simulink model "kers_discharge_22_6_update_2019a"  (R2019b)
settings: Solver=ode4  StartTime=0.0  StopTime=50  FixedStep=0.01  RelTol=1e-3
values from neighbouring files (symbols this model uses):
  d = 0.5*rho*Cx*Sf    (= 0.81)    [Data.m]
  Jeq_v = M*Rw^2    (= 83.853)    [Data.m]
  Jf = 1/2*(Rf^2*Mf)    (= 0.025)    [Data.m]
  k = 4/3*mi_d*R_clutch    (= 0.096)    [Data.m]
  Rw = 0.33    [Data.m]
  tau1 = 1/3.08    (= 0.324675324675)    [Data.m]
  tau2 = 1/2.18    (= 0.45871559633)    [Data.m]
  tau3 = 1/1.63    (= 0.613496932515)    [Data.m]
  tau4 = 1/1.29    (= 0.77519379845)    [Data.m]
  tau5 = 1/1.03    (= 0.970873786408)    [Data.m]
  tau6 = 1/0.84    (= 1.19047619048)    [Data.m]
  tau7 = 1/0.69    (= 1.44927536232)    [Data.m]
  tau_max = 2.5    [Data.m]
  tau_min = 0.4    [Data.m]
  tau_trasm_discharge = 1/(tauk_discharge*tauf)    (= 4.77818181818)    [Data.m]
  tauf = 1/4.38    (= 0.228310502283)    [Data.m]
  tauk_discharge = 11*tauk_charge    (= 0.916666666667)    [Data.m]
  Tmax = 240    [Data.m]
  V1max = tauf*tau1*Rw*Wmax    (= 23.0528375734)    [Data.m]
  V2max = tauf*tau2*Rw*Wmax    (= 32.5700640945)    [Data.m]
  V3max = tauf*tau3*Rw*Wmax    (= 43.5599630221)    [Data.m]
  V4max = tauf*tau4*Rw*Wmax    (= 55.0408835085)    [Data.m]
  V5max = tauf*tau5*Rw*Wmax    (= 68.9346987631)    [Data.m]
  V6max = tauf*tau6*Rw*Wmax    (= 84.5270711024)    [Data.m]
  wf_max = 64500/9.55    (= 6753.92670157)    [Data.m]
libraries: simulink x3
settings Model: Creator=andre  LastModifiedBy=andre
settings SolverCC: ZeroCrossControl=DisableAll
settings SFSimCC: CustomCodeUndefinedFunction=UseInterfaceOnly

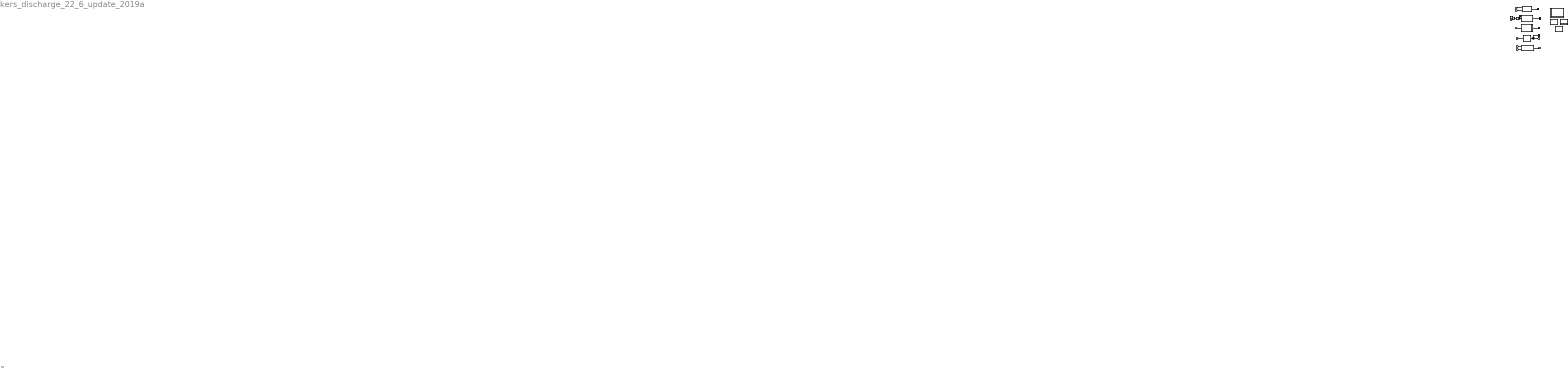
== system kers_discharge_22_6_update_2019a ==
  note: KERS DISCHARGE
  note: v [km/h]
  note: w_f [rpm]
  note: v [km/h]
  note: tau
  Compute Force control for clutch engagement : Subsystem
  Compute Paero : Subsystem
  Compute Pclutch : Subsystem
  Compute Torque to the wheels : Subsystem
  Constant : Constant  Value=Tmax  SampleTime=-1
  From6 : From  Commented=on  GotoTag=Teq  TagVisibility=global
  GearBox : Subsystem
      mask Display: image("GearBox.jpg")
  KERS : Subsystem
      mask Display: image('KERS.jpg'); % Use "Edit Image" on toolstrip to change.
  Product : Product
  Scope{,1..4} (5 alike) : Scope
  Torotrak : Subsystem
      mask Display: image('Torotrak.jpg'); % Use "Edit Image" on toolstrip to change.
  Torque ICE : Subsystem
      mask Display: image("ICE.jpg")
  Vehicle Dynamics : Subsystem
      mask Display: image('Ferrari.jpg'); % Use "Edit Image" on toolstrip to change.
  tag scope: Te=global, taugb=global
  wires:
  [wr] -> Torotrak/1(In1)
  [wf] -> Torotrak/2(In2)
  Torotrak/1(Out1) -> Scope3/1
  [Teq] -> Vehicle Dynamics/1(In1)
  Vehicle Dynamics/1(Out1) -> Scope/1
  KERS/1(Out1) -> Scope1/1
  [v] -> GearBox/1(In1)
  GearBox/1(Out1) -> [taugb], Scope2/1
  [v] -> Torque ICE/1(In1)
  [taugb] -> Torque ICE/2(In2)
  Torque ICE/1(Out1) -> [Te]
  Product/1 -> Scope4/1, KERS/1(In1)
  Constant/1 -> Product/1
  [logic] -> Product/2

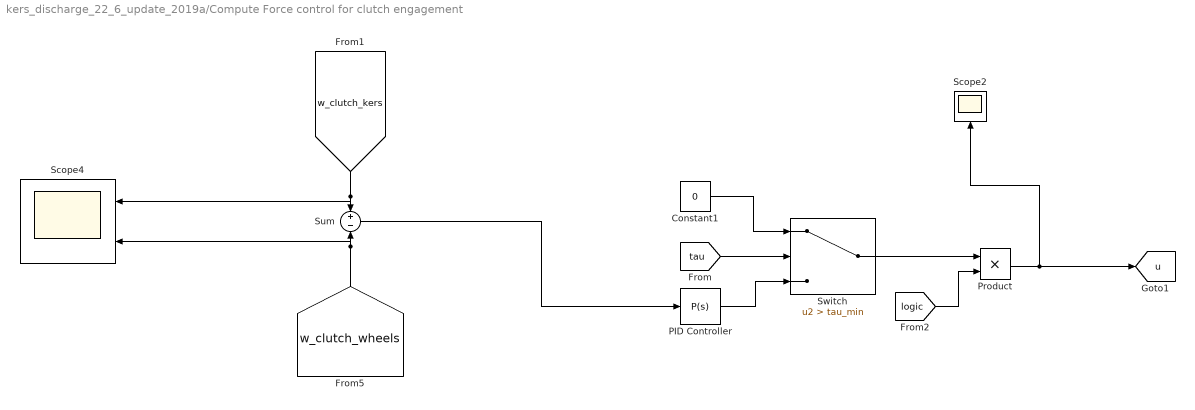
== system kers_discharge_22_6_update_2019a/Compute Force control for clutch engagement ==
  Constant1 : Constant  Value=0  SampleTime=-1
  PID Controller : simulink/Continuous/PID Controller  Controller=P  Form=Parallel  TimeDomain=Continuous-time  SampleTime=-1  IntegratorMethod=Forward Euler  FilterMethod=Forward Euler  ControllerParametersSource=internal  P=0.5  I=1  D=4  UseFilter=on  N=100  TunerSelectOption=Transfer Function Based (PID Tuner App)  InitialConditionSource=internal  InitialConditionForIntegrator=0  InitialConditionForFilter=0  DifferentiatorICPrevScaledInput=0  ExternalReset=none  TrackingMode=off  Kt=1  LimitOutput=off  UpperSaturationLimit=inf  LowerSaturationLimit=-inf  LinearizeAsGain=on  AntiWindupMode=none  Kb=1  POutMin=[]  POutMax=[]  IOutMin=[]  IOutMax=[]  DOutMin=[]  DOutMax=[]  NOutMin=[]  NOutMax=[]  SumOutMin=[]  SumOutMax=[]  SaturationOutMin=[]  SaturationOutMax=[]  PParamMin=[]  PParamMax=[]  IParamMin=[]  IParamMax=[]  DParamMin=[]  DParamMax=[]  NParamMin=[]  NParamMax=[]  KbParamMin=[]  KbParamMax=[]  KtParamMin=[]  KtParamMax=[]  KbOutMin=[]  KbOutMax=[]  KtOutMin=[]  KtOutMax=[]  IntegratorOutMin=[]  IntegratorOutMax=[]  FilterOutMin=[]  FilterOutMax=[]  SumI1OutMin=[]  SumI1OutMax=[]  SumI2OutMin=[]  SumI2OutMax=[]  SumI3OutMin=[]  SumI3OutMax=[]  SumI4OutMin=[]  SumI4OutMax=[]  SumDOutMin=[]  SumDOutMax=[]  DifferentiatorOutMin=[]  DifferentiatorOutMax=[]  FilterDiffOutCoefMin=[]  FilterDiffOutCoefMax=[]  ReciprocalOutMin=[]  ReciprocalOutMax=[]  SumDenOutMin=[]  SumDenOutMax=[]  SumNumOutMin=[]  SumNumOutMax=[]  DivideOutMin=[]  DivideOutMax=[]  IntegratorContinuousStateAttributes=''  IntegratorStateMustResolveToSignalObject=off  IntegratorRTWStateStorageClass=Auto  FilterContinuousStateAttributes=''  FilterStateMustResolveToSignalObject=off  FilterRTWStateStorageClass=Auto  ParallelPVariant=InternalParameters  IdealPVariant=Disabled  IVariant=Disabled  DVariant=Disabled  IntegratorVariant=Disabled  SatVariant=Disabled  AWVariant=Disabled  PCopyVariant=Disabled  TRVariant=Disabled  FdbkBlocksVariant=Forward  IdealPFdbkVariant=Disabled  SatFdbkVariant=Disabled  DerivativeFilterVariant=Disabled  NVariant=Disabled  NCopyVariant=Disabled_SignalSpec  FilterICVariant=Disabled  IntegratorICVariant=Disabled  ExternalResetVariant=Disabled  TRSumVariant=Passthrough  SumFdbkVariant=Disabled  SumVariant=Passthrough_P
  Product : Product
  Scope2 : Scope
  Scope4 : Scope  NumInputPorts=2
  Sum : Sum  Inputs=+-
  Switch : Switch  Criteria=u2 > Threshold  Threshold=tau_min
  tag scope: u=global
  wires:
  [tau] -> Switch/2
  [w_clutch_kers] -> Scope4/1, Sum/1
  [w_clutch_wheels] -> Scope4/2, Sum/2
  Constant1/1 -> Switch/1
  PID Controller/1 -> Switch/3
  Switch/1 -> Product/1
  [logic] -> Product/2
  Product/1 -> Scope2/1, [u]
  Sum/1 -> PID Controller/1

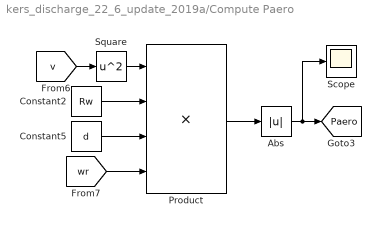
== system kers_discharge_22_6_update_2019a/Compute Paero ==
  Abs : Abs  ZeroCross=off
  Constant2 : Constant  Value=Rw
  Constant5 : Constant  Value=d
  Product : Product  Inputs=4
  Scope : Scope
  Square : Math  Operator=square  SignedPower=on  SaturateOnIntegerOverflow=on
  tag scope: Paero=global
  wires:
  Square/1 -> Product/1
  Constant5/1 -> Product/3
  [wr] -> Product/4
  [v] -> Square/1
  Constant2/1 -> Product/2
  Product/1 -> Abs/1
  Abs/1 -> Scope/1, [Paero]

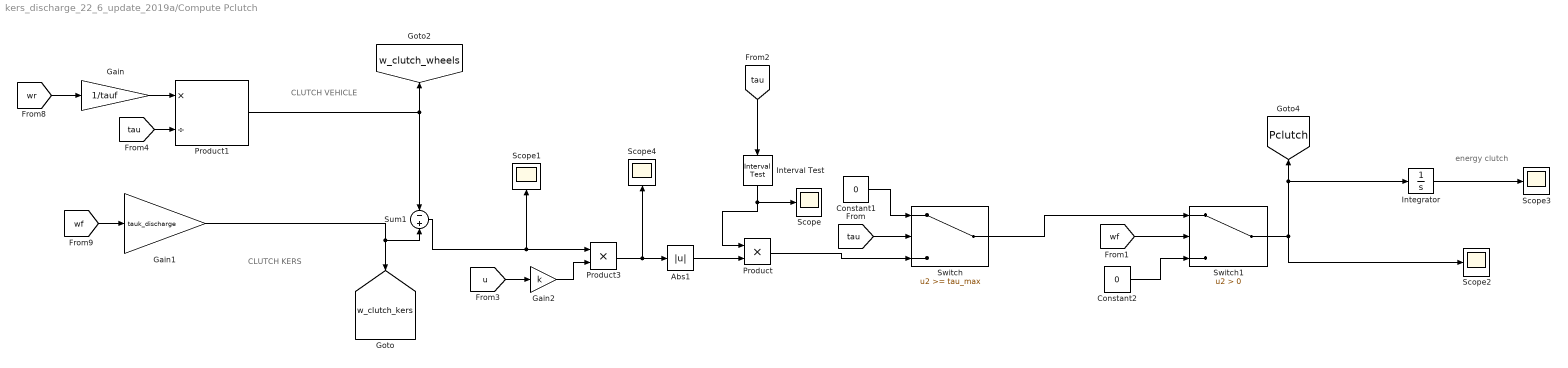
== system kers_discharge_22_6_update_2019a/Compute Pclutch ==
  note: energy clutch
  note: CLUTCH VEHICLE
  note: CLUTCH KERS
  Abs1 : Abs  ZeroCross=off
  Constant1 : Constant  Value=0
  Constant2 : Constant  Value=0
  Gain : Gain  Gain=1/tauf
  Gain1 : Gain  Gain=tauk_discharge
  Gain2 : Gain  Gain=k
  Integrator : Integrator
  Interval Test : simulink/Logic and Bit Operations/Interval Test  IntervalClosedRight=on  uplimit=2.49  IntervalClosedLeft=on  lowlimit=tau_min  OutDataTypeStr=boolean
  Product : Product
  Product1 : Product  Inputs=*/
  Product3 : Product
  Scope{,1..4} (5 alike) : Scope
  Sum1 : Sum  Inputs=-+
  Switch : Switch  Threshold=tau_max  ZeroCross=off
  Switch1 : Switch  Criteria=u2 > Threshold  ZeroCross=off
  tag scope: Pclutch=global, w_clutch_kers=global, w_clutch_wheels=global
  wires:
  Sum1/1 -> Scope1/1, Product3/1
  Product3/1 -> Scope4/1, Abs1/1
  [tau] -> Switch/2
  [wf] -> Switch1/2
  Integrator/1 -> Scope3/1
  Switch1/1 -> Scope2/1, Integrator/1, [Pclutch]
  Constant1/1 -> Switch/1
  Switch/1 -> Switch1/1
  Constant2/1 -> Switch1/3
  Abs1/1 -> Product/2
  [tau] -> Interval Test/1
  Product/1 -> Switch/3
  Interval Test/1 -> Product/1, Scope/1
  [tau] -> Product1/2
  Product1/1 -> [w_clutch_wheels], Sum1/1
  [wf] -> Gain1/1
  [wr] -> Gain/1
  Gain1/1 -> [w_clutch_kers], Sum1/2
  Gain/1 -> Product1/1
  [u] -> Gain2/1
  Gain2/1 -> Product3/2

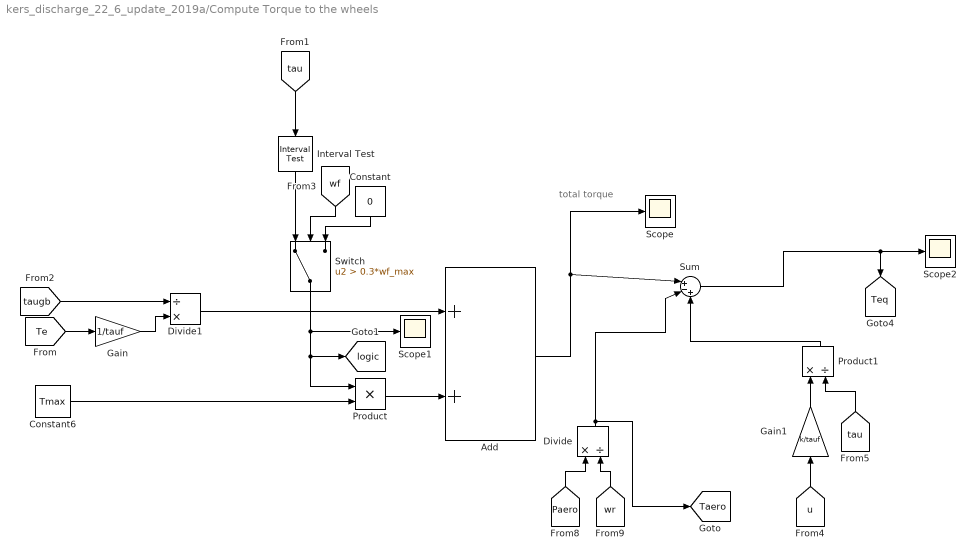
== system kers_discharge_22_6_update_2019a/Compute Torque to the wheels ==
  note: total torque
  Add : Sum
  Constant : Constant  Value=0  SampleTime=-1
  Constant6 : Constant  Value=Tmax
  Divide : Product  Inputs=*/
  Divide1 : Product  Inputs=/*
  Gain : Gain  Gain=1/tauf
  Gain1 : Gain  Gain=k/tauf
  Interval Test : simulink/Logic and Bit Operations/Interval Test  IntervalClosedRight=off  uplimit=tau_max  IntervalClosedLeft=on  lowlimit=tau_min  OutDataTypeStr=boolean
  Product : Product
  Product1 : Product  Inputs=*/
  Scope : Scope
  Scope1 : Scope
  Scope2 : Scope
  Sum : Sum  Inputs=|+-+
  Switch : Switch  Criteria=u2 > Threshold  Threshold=0.3*wf_max
  tag scope: Taero=global, Teq=global, logic=global
  wires:
  Sum/1 -> [Teq], Scope2/1
  [Paero] -> Divide/1
  [wr] -> Divide/2
  Divide/1 -> Sum/2, [Taero]
  [Te] -> Gain/1
  Gain/1 -> Divide1/2
  [taugb] -> Divide1/1
  Constant6/1 -> Product/2
  [tau] -> Interval Test/1
  Interval Test/1 -> Switch/1
  Product/1 -> Add/2
  Add/1 -> Scope/1, Sum/1
  Constant/1 -> Switch/3
  [wf] -> Switch/2
  Switch/1 -> Scope1/1, [logic], Product/1
  Divide1/1 -> Add/1
  [u] -> Gain1/1
  Product1/1 -> Sum/3
  Gain1/1 -> Product1/1
  [tau] -> Product1/2

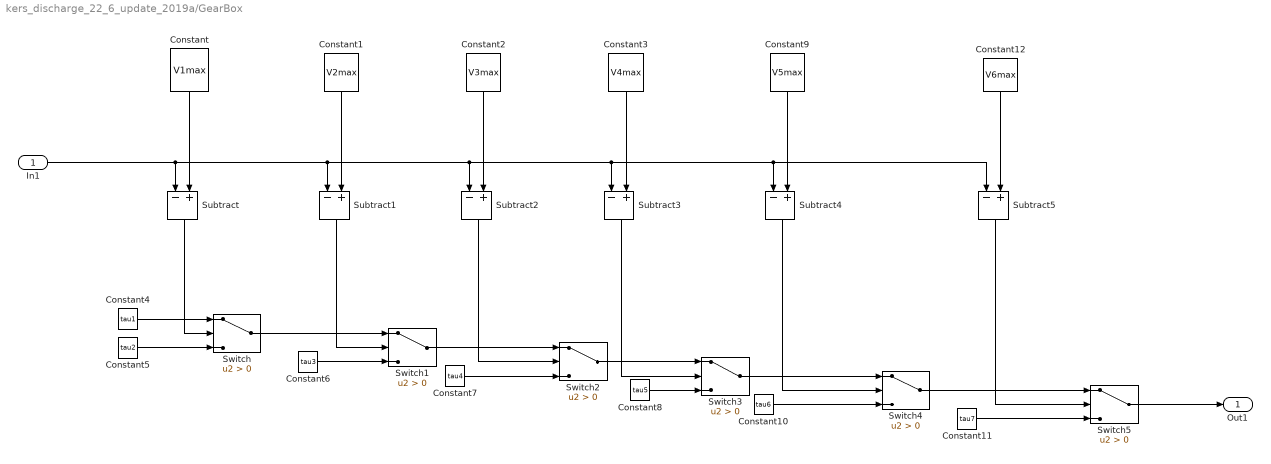
== system kers_discharge_22_6_update_2019a/GearBox ==
  In1 : Inport
  Constant : Constant  Value=V1max
  Constant1 : Constant  Value=V2max
  Constant10 : Constant  Value=tau6
  Constant11 : Constant  Value=tau7
  Constant12 : Constant  Value=V6max
  Constant2 : Constant  Value=V3max
  Constant3 : Constant  Value=V4max
  Constant4 : Constant  Value=tau1
  Constant5 : Constant  Value=tau2
  Constant6 : Constant  Value=tau3
  Constant7 : Constant  Value=tau4
  Constant8 : Constant  Value=tau5
  Constant9 : Constant  Value=V5max
  Subtract{,1..5} (6 alike) : Sum  Inputs=-+
  Switch{,1..5} (6 alike) : Switch  Criteria=u2 > Threshold
  Out1 : Outport  VectorParamsAs1DForOutWhenUnconnected=off
  wires:
  Constant/1 -> Subtract/2
  In1/1 -> Subtract/1, Subtract1/1, Subtract2/1, Subtract3/1, Subtract4/1, Subtract5/1
  Constant1/1 -> Subtract1/2
  Constant2/1 -> Subtract2/2
  Constant3/1 -> Subtract3/2
  Subtract/1 -> Switch/2
  Constant4/1 -> Switch/1
  Constant5/1 -> Switch/3
  Subtract1/1 -> Switch1/2
  Switch/1 -> Switch1/1
  Constant6/1 -> Switch1/3
  Switch1/1 -> Switch2/1
  Subtract2/1 -> Switch2/2
  Constant7/1 -> Switch2/3
  Switch2/1 -> Switch3/1
  Subtract3/1 -> Switch3/2
  Constant8/1 -> Switch3/3
  Constant9/1 -> Subtract4/2
  Subtract4/1 -> Switch4/2
  Switch3/1 -> Switch4/1
  Constant10/1 -> Switch4/3
  Constant11/1 -> Switch5/3
  Constant12/1 -> Subtract5/2
  Subtract5/1 -> Switch5/2
  Switch4/1 -> Switch5/1
  Switch5/1 -> Out1/1

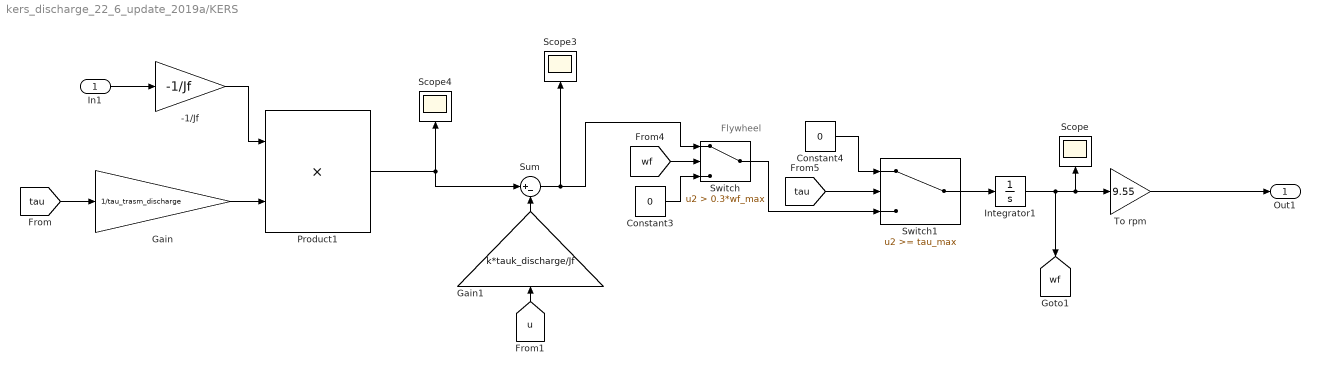
== system kers_discharge_22_6_update_2019a/KERS ==
  note: Flywheel
  In1 : Inport
  -1/Jf : Gain  Gain=-1/Jf
  Constant3 : Constant  Value=0
  Constant4 : Constant  Value=0
  Gain : Gain  Gain=1/tau_trasm_discharge
  Gain1 : Gain  Gain=k*tauk_discharge/Jf
  Integrator1 : Integrator  InitialCondition=wf_max  ContinuousStateAttributes="\"omega_f\""
  Product1 : Product  Inputs=**
  Scope : Scope
  Scope3 : Scope
  Scope4 : Scope
  Sum : Sum  Inputs=|+-
  Switch : Switch  Criteria=u2 > Threshold  Threshold=0.3*wf_max
  Switch1 : Switch  Threshold=tau_max
  To rpm : Gain  Gain=9.55
  Out1 : Outport
  tag scope: wf=global
  wires:
  Switch1/1 -> Integrator1/1
  -1/Jf/1 -> Product1/1
  Integrator1/1 -> Scope/1, To rpm/1, [wf]
  [wf] -> Switch/2
  [tau] -> Switch1/2
  Product1/1 -> Sum/1, Scope4/1
  To rpm/1 -> Out1/1
  In1/1 -> -1/Jf/1
  Gain/1 -> Product1/2
  [tau] -> Gain/1
  Constant3/1 -> Switch/3
  Constant4/1 -> Switch1/1
  Switch/1 -> Switch1/3
  Sum/1 -> Switch/1, Scope3/1
  [u] -> Gain1/1
  Gain1/1 -> Sum/2

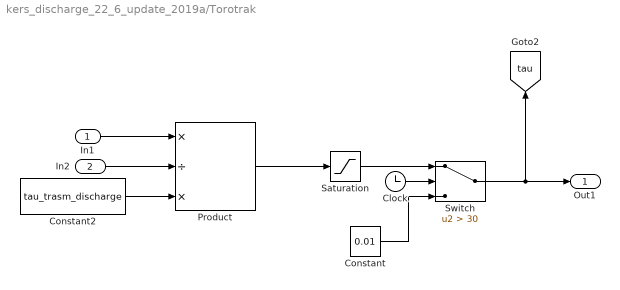
== system kers_discharge_22_6_update_2019a/Torotrak ==
  In1 : Inport
  In2 : Inport  Port=2
  Clock : Clock
  Constant : Constant  Value=0.01  SampleTime=-1
  Constant2 : Constant  Value=tau_trasm_discharge
  Product : Product  Inputs=*/*
  Saturation : Saturate  UpperLimit=tau_max  LowerLimit=tau_min  ZeroCross=off
  Switch : Switch  Criteria=u2 > Threshold  Threshold=30  ZeroCross=off
  Out1 : Outport
  tag scope: tau=global
  wires:
  In2/1 -> Product/2
  Constant2/1 -> Product/3
  In1/1 -> Product/1
  Product/1 -> Saturation/1
  Switch/1 -> [tau], Out1/1
  Saturation/1 -> Switch/1
  Constant/1 -> Switch/3
  Clock/1 -> Switch/2

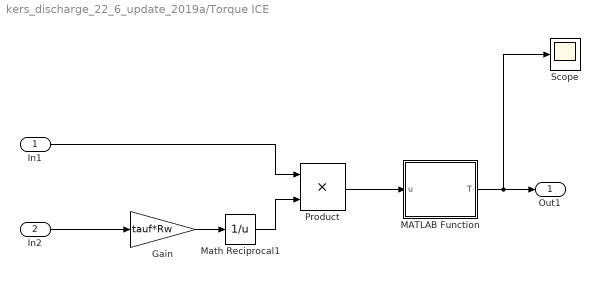
== system kers_discharge_22_6_update_2019a/Torque ICE ==
  In1 : Inport
  In2 : Inport  Port=2
  Gain : Gain  Gain=tauf*Rw
  MATLAB Function : MATLAB Function  TreatAsAtomicUnit=on
  Math Reciprocal1 : Math  Operator=reciprocal  SignedPower=on  SaturateOnIntegerOverflow=on
  Product : Product
  Scope : Scope
  Out1 : Outport  VectorParamsAs1DForOutWhenUnconnected=off
  wires:
  In2/1 -> Gain/1
  Gain/1 -> Math Reciprocal1/1
  Math Reciprocal1/1 -> Product/2
  In1/1 -> Product/1
  MATLAB Function/1(T) -> Scope/1, Out1/1
  Product/1 -> MATLAB Function/1(u)

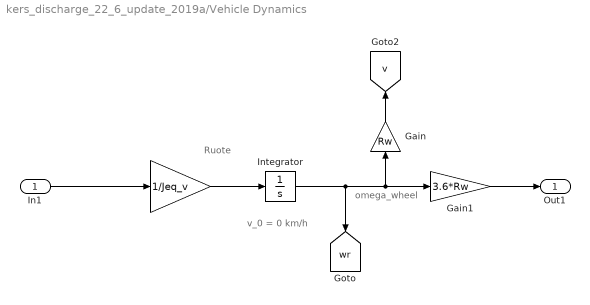
== system kers_discharge_22_6_update_2019a/Vehicle Dynamics ==
  note: omega_wheel
  note: v_0 = 0 km/h
  note: Ruote
  In1 : Inport
  " " : Gain  Gain=1/Jeq_v
  Gain : Gain  Gain=Rw
  Gain1 : Gain  Gain=3.6*Rw
  Integrator : Integrator  InitialCondition=0.0000001/(3.6*Rw)  ContinuousStateAttributes="\"omega_w\""
  Out1 : Outport
  tag scope: v=global, wr=global
  wires:
  Integrator/1 -> Gain/1, Gain1/1, [wr]
  In1/1 -> " "/1
  Gain/1 -> [v]
  " "/1 -> Integrator/1
  Gain1/1 -> Out1/1

== matlab function kers_discharge_22_6_update_2019a/Torque ICE/MATLAB Function ==
  data: u input; T output
function T = TorqueICE(u)

a0 = 88.48;
a1 = 1.41;
a2 = -8.36e-4;

T = a0+a1*u+a2*(u^2);
